simulink model "FunctionalArchitecture"  (R2020b)
settings: Solver=VariableStepAuto  StartTime=0.0  StopTime=10.0  RelTol=1e-3
settings Model: Creator=jantonio  LastModifiedBy=jantonio

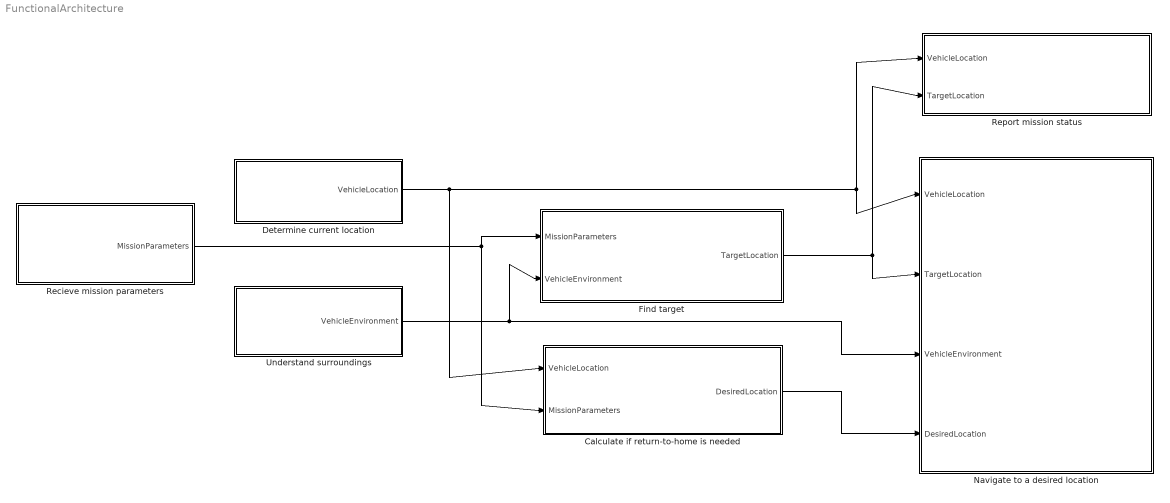
== system FunctionalArchitecture ==
  Calculate if return-to-home is needed : Subsystem
      settings: PortSchema="{\"entries\":[{\"content\":{\"headerSize\":26,\"margin\":15,\"minimumSpacing\":25,\"sides\":[{\"content\":{\"connectorIds\":[\"In2\",\"In1\"]},\"type\":\"ConnectorPlacement.EquallySpacedRectSide\",\"uuid\":\"39ab5f6e-200b-418c-957c-0427e0a2d192\"},{\"content\":{\"connectorIds\":[\"Out1\"],\"side\":\"RIGHT\"},\"type\":\"ConnectorPlacement.EquallySpacedRectSide\",\"uuid\":\"2abcd6b7-9ef0-4689-b904-6f1a8a48cdb7\"},{\"content\":{\"connectorIds\":[],\"side\":\"TOP\"},\"type\":\"ConnectorPlacement.EquallySpacedRectSide\",\"uuid\":\"3ddcf8bd-fb65-4c69-ae6b-4c30928b7beb\"}]},\"type\":\"ConnectorPlacement.EquallySpacedConnector\",\"uuid\":\"ab0c7103-d8ef-4055-8653-3cf105b5edbd\"}],\"packageUris\":[\"http://schema.mathworks.com/mf0/Connector/19700101\"],\"version\":\"1.0\"}"
  Determine current location : Subsystem
      settings: PortSchema="{\"entries\":[{\"content\":{\"headerSize\":26,\"margin\":15,\"minimumSpacing\":25,\"sides\":[{\"content\":{\"connectorIds\":[]},\"type\":\"ConnectorPlacement.EquallySpacedRectSide\",\"uuid\":\"39ab5f6e-200b-418c-957c-0427e0a2d192\"},{\"content\":{\"connectorIds\":[\"Out1\"],\"side\":\"RIGHT\"},\"type\":\"ConnectorPlacement.EquallySpacedRectSide\",\"uuid\":\"2abcd6b7-9ef0-4689-b904-6f1a8a48cdb7\"},{\"content\":{\"connectorIds\":[],\"side\":\"TOP\"},\"type\":\"ConnectorPlacement.EquallySpacedRectSide\",\"uuid\":\"3ddcf8bd-fb65-4c69-ae6b-4c30928b7beb\"}]},\"type\":\"ConnectorPlacement.EquallySpacedConnector\",\"uuid\":\"ab0c7103-d8ef-4055-8653-3cf105b5edbd\"}],\"packageUris\":[\"http://schema.mathworks.com/mf0/Connector/19700101\"],\"version\":\"1.0\"}"
  Find target : Subsystem
      settings: PortSchema="{\"entries\":[{\"content\":{\"headerSize\":26,\"margin\":15,\"minimumSpacing\":25,\"sides\":[{\"content\":{\"connectorIds\":[\"In1\",\"In2\"]},\"type\":\"ConnectorPlacement.EquallySpacedRectSide\",\"uuid\":\"39ab5f6e-200b-418c-957c-0427e0a2d192\"},{\"content\":{\"connectorIds\":[\"Out1\"],\"side\":\"RIGHT\"},\"type\":\"ConnectorPlacement.EquallySpacedRectSide\",\"uuid\":\"2abcd6b7-9ef0-4689-b904-6f1a8a48cdb7\"},{\"content\":{\"connectorIds\":[],\"side\":\"TOP\"},\"type\":\"ConnectorPlacement.EquallySpacedRectSide\",\"uuid\":\"3ddcf8bd-fb65-4c69-ae6b-4c30928b7beb\"}]},\"type\":\"ConnectorPlacement.EquallySpacedConnector\",\"uuid\":\"ab0c7103-d8ef-4055-8653-3cf105b5edbd\"}],\"packageUris\":[\"http://schema.mathworks.com/mf0/Connector/19700101\"],\"version\":\"1.0\"}"
  Navigate to a desired location : Subsystem
      settings: PortSchema="{\"entries\":[{\"content\":{\"headerSize\":26,\"margin\":15,\"minimumSpacing\":25,\"sides\":[{\"content\":{\"connectorIds\":[\"In3\",\"In2\",\"In4\",\"In1\"]},\"type\":\"ConnectorPlacement.EquallySpacedRectSide\",\"uuid\":\"39ab5f6e-200b-418c-957c-0427e0a2d192\"},{\"content\":{\"connectorIds\":[],\"side\":\"RIGHT\"},\"type\":\"ConnectorPlacement.EquallySpacedRectSide\",\"uuid\":\"2abcd6b7-9ef0-4689-b904-6f1a8a48cdb7\"},{\"content\":{\"connectorIds\":[],\"side\":\"TOP\"},\"type\":\"ConnectorPlacement.EquallySpacedRectSide\",\"uuid\":\"3ddcf8bd-fb65-4c69-ae6b-4c30928b7beb\"}]},\"type\":\"ConnectorPlacement.EquallySpacedConnector\",\"uuid\":\"ab0c7103-d8ef-4055-8653-3cf105b5edbd\"}],\"packageUris\":[\"http://schema.mathworks.com/mf0/Connector/19700101\"],\"version\":\"1.0\"}"
  Recieve mission parameters : Subsystem
      settings: PortSchema="{\"entries\":[{\"content\":{\"headerSize\":26,\"margin\":15,\"minimumSpacing\":25,\"sides\":[{\"content\":{\"connectorIds\":[]},\"type\":\"ConnectorPlacement.EquallySpacedRectSide\",\"uuid\":\"39ab5f6e-200b-418c-957c-0427e0a2d192\"},{\"content\":{\"connectorIds\":[\"Out1\"],\"side\":\"RIGHT\"},\"type\":\"ConnectorPlacement.EquallySpacedRectSide\",\"uuid\":\"2abcd6b7-9ef0-4689-b904-6f1a8a48cdb7\"},{\"content\":{\"connectorIds\":[],\"side\":\"TOP\"},\"type\":\"ConnectorPlacement.EquallySpacedRectSide\",\"uuid\":\"3ddcf8bd-fb65-4c69-ae6b-4c30928b7beb\"}]},\"type\":\"ConnectorPlacement.EquallySpacedConnector\",\"uuid\":\"ab0c7103-d8ef-4055-8653-3cf105b5edbd\"}],\"packageUris\":[\"http://schema.mathworks.com/mf0/Connector/19700101\"],\"version\":\"1.0\"}"
  Report mission status : Subsystem
      settings: PortSchema="{\"entries\":[{\"content\":{\"headerSize\":26,\"margin\":15,\"minimumSpacing\":25,\"sides\":[{\"content\":{\"connectorIds\":[\"In2\",\"In1\"]},\"type\":\"ConnectorPlacement.EquallySpacedRectSide\",\"uuid\":\"39ab5f6e-200b-418c-957c-0427e0a2d192\"},{\"content\":{\"connectorIds\":[],\"side\":\"RIGHT\"},\"type\":\"ConnectorPlacement.EquallySpacedRectSide\",\"uuid\":\"2abcd6b7-9ef0-4689-b904-6f1a8a48cdb7\"},{\"content\":{\"connectorIds\":[],\"side\":\"TOP\"},\"type\":\"ConnectorPlacement.EquallySpacedRectSide\",\"uuid\":\"3ddcf8bd-fb65-4c69-ae6b-4c30928b7beb\"}]},\"type\":\"ConnectorPlacement.EquallySpacedConnector\",\"uuid\":\"ab0c7103-d8ef-4055-8653-3cf105b5edbd\"}],\"packageUris\":[\"http://schema.mathworks.com/mf0/Connector/19700101\"],\"version\":\"1.0\"}"
  Understand surroundings : Subsystem
      settings: PortSchema="{\"entries\":[{\"content\":{\"headerSize\":26,\"margin\":15,\"minimumSpacing\":25,\"sides\":[{\"content\":{\"connectorIds\":[]},\"type\":\"ConnectorPlacement.EquallySpacedRectSide\",\"uuid\":\"39ab5f6e-200b-418c-957c-0427e0a2d192\"},{\"content\":{\"connectorIds\":[\"Out1\"],\"side\":\"RIGHT\"},\"type\":\"ConnectorPlacement.EquallySpacedRectSide\",\"uuid\":\"2abcd6b7-9ef0-4689-b904-6f1a8a48cdb7\"},{\"content\":{\"connectorIds\":[],\"side\":\"TOP\"},\"type\":\"ConnectorPlacement.EquallySpacedRectSide\",\"uuid\":\"3ddcf8bd-fb65-4c69-ae6b-4c30928b7beb\"}]},\"type\":\"ConnectorPlacement.EquallySpacedConnector\",\"uuid\":\"ab0c7103-d8ef-4055-8653-3cf105b5edbd\"}],\"packageUris\":[\"http://schema.mathworks.com/mf0/Connector/19700101\"],\"version\":\"1.0\"}"
  wires:
  Find target/1(TargetLocation) -> Report mission status/1(TargetLocation), Navigate to a desired location/2(TargetLocation)
  Understand surroundings/1(VehicleEnvironment) -> Find target/2(VehicleEnvironment), Navigate to a desired location/4(VehicleEnvironment)
  Determine current location/1(VehicleLocation) -> Calculate if return-to-home is needed/2(VehicleLocation), Report mission status/2(VehicleLocation), Navigate to a desired location/3(VehicleLocation)
  Recieve mission parameters/1(MissionParameters) -> Calculate if return-to-home is needed/1(MissionParameters), Find target/1(MissionParameters)
  Calculate if return-to-home is needed/1(DesiredLocation) -> Navigate to a desired location/1(DesiredLocation)

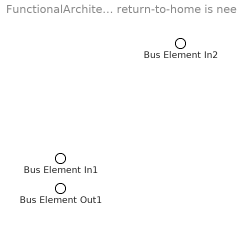
== system FunctionalArchitecture/Calculate if return-to-home is needed ==
  Bus Element In2 : Inport  PortName=MissionParameters
  Bus Element In1 : Inport  Port=2  PortName=VehicleLocation
  Bus Element Out1 : Outport  PortName=DesiredLocation

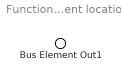
== system FunctionalArchitecture/Determine current location ==
  Bus Element Out1 : Outport  PortName=VehicleLocation

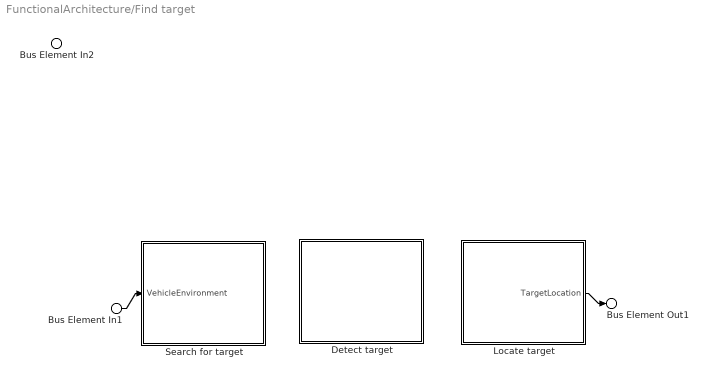
== system FunctionalArchitecture/Find target ==
  Bus Element In2 : Inport  PortName=MissionParameters
  Bus Element In1 : Inport  Port=2  PortName=VehicleEnvironment
  Detect target : Subsystem
      settings: PortSchema="{\"entries\":[{\"content\":{\"headerSize\":26,\"margin\":15,\"minimumSpacing\":25,\"sides\":[{\"content\":{\"connectorIds\":[]},\"type\":\"ConnectorPlacement.EquallySpacedRectSide\",\"uuid\":\"39ab5f6e-200b-418c-957c-0427e0a2d192\"},{\"content\":{\"connectorIds\":[],\"side\":\"RIGHT\"},\"type\":\"ConnectorPlacement.EquallySpacedRectSide\",\"uuid\":\"2abcd6b7-9ef0-4689-b904-6f1a8a48cdb7\"},{\"content\":{\"connectorIds\":[],\"side\":\"TOP\"},\"type\":\"ConnectorPlacement.EquallySpacedRectSide\",\"uuid\":\"3ddcf8bd-fb65-4c69-ae6b-4c30928b7beb\"}]},\"type\":\"ConnectorPlacement.EquallySpacedConnector\",\"uuid\":\"ab0c7103-d8ef-4055-8653-3cf105b5edbd\"}],\"packageUris\":[\"http://schema.mathworks.com/mf0/Connector/19700101\"],\"version\":\"1.0\"}"
  Locate target : Subsystem
      settings: PortSchema="{\"entries\":[{\"content\":{\"headerSize\":26,\"margin\":15,\"minimumSpacing\":25,\"sides\":[{\"content\":{\"connectorIds\":[]},\"type\":\"ConnectorPlacement.EquallySpacedRectSide\",\"uuid\":\"39ab5f6e-200b-418c-957c-0427e0a2d192\"},{\"content\":{\"connectorIds\":[\"Out1\"],\"side\":\"RIGHT\"},\"type\":\"ConnectorPlacement.EquallySpacedRectSide\",\"uuid\":\"2abcd6b7-9ef0-4689-b904-6f1a8a48cdb7\"},{\"content\":{\"connectorIds\":[],\"side\":\"TOP\"},\"type\":\"ConnectorPlacement.EquallySpacedRectSide\",\"uuid\":\"3ddcf8bd-fb65-4c69-ae6b-4c30928b7beb\"}]},\"type\":\"ConnectorPlacement.EquallySpacedConnector\",\"uuid\":\"ab0c7103-d8ef-4055-8653-3cf105b5edbd\"}],\"packageUris\":[\"http://schema.mathworks.com/mf0/Connector/19700101\"],\"version\":\"1.0\"}"
  Search for target : Subsystem
      settings: PortSchema="{\"entries\":[{\"content\":{\"headerSize\":26,\"margin\":15,\"minimumSpacing\":25,\"sides\":[{\"content\":{\"connectorIds\":[\"In1\"]},\"type\":\"ConnectorPlacement.EquallySpacedRectSide\",\"uuid\":\"39ab5f6e-200b-418c-957c-0427e0a2d192\"},{\"content\":{\"connectorIds\":[],\"side\":\"RIGHT\"},\"type\":\"ConnectorPlacement.EquallySpacedRectSide\",\"uuid\":\"2abcd6b7-9ef0-4689-b904-6f1a8a48cdb7\"},{\"content\":{\"connectorIds\":[],\"side\":\"TOP\"},\"type\":\"ConnectorPlacement.EquallySpacedRectSide\",\"uuid\":\"3ddcf8bd-fb65-4c69-ae6b-4c30928b7beb\"}]},\"type\":\"ConnectorPlacement.EquallySpacedConnector\",\"uuid\":\"ab0c7103-d8ef-4055-8653-3cf105b5edbd\"}],\"packageUris\":[\"http://schema.mathworks.com/mf0/Connector/19700101\"],\"version\":\"1.0\"}"
  Bus Element Out1 : Outport  PortName=TargetLocation
  wires:
  Bus Element In1/1 -> Search for target/1(VehicleEnvironment)
  Locate target/1(TargetLocation) -> Bus Element Out1/1

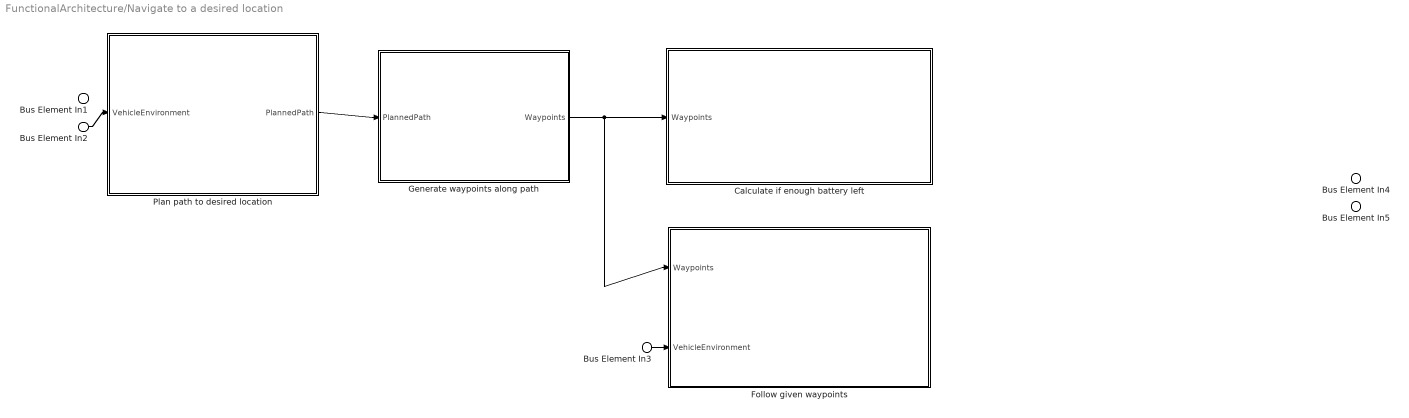
== system FunctionalArchitecture/Navigate to a desired location ==
  Bus Element In5 : Inport  PortName=DesiredLocation
  Bus Element In1 : Inport  Port=2  PortName=TargetLocation
  Bus Element In4 : Inport  Port=3  PortName=VehicleLocation
  Bus Element In3 : Inport  Port=4  PortName=VehicleEnvironment
  Bus Element In2 : Inport  Port=4  PortName=VehicleEnvironment
  Calculate if enough battery left : Subsystem
      settings: PortSchema="{\"entries\":[{\"content\":{\"headerSize\":26,\"margin\":15,\"minimumSpacing\":25,\"sides\":[{\"content\":{\"connectorIds\":[\"In1\"]},\"type\":\"ConnectorPlacement.EquallySpacedRectSide\",\"uuid\":\"39ab5f6e-200b-418c-957c-0427e0a2d192\"},{\"content\":{\"connectorIds\":[],\"side\":\"RIGHT\"},\"type\":\"ConnectorPlacement.EquallySpacedRectSide\",\"uuid\":\"2abcd6b7-9ef0-4689-b904-6f1a8a48cdb7\"},{\"content\":{\"connectorIds\":[],\"side\":\"TOP\"},\"type\":\"ConnectorPlacement.EquallySpacedRectSide\",\"uuid\":\"3ddcf8bd-fb65-4c69-ae6b-4c30928b7beb\"}]},\"type\":\"ConnectorPlacement.EquallySpacedConnector\",\"uuid\":\"ab0c7103-d8ef-4055-8653-3cf105b5edbd\"}],\"packageUris\":[\"http://schema.mathworks.com/mf0/Connector/19700101\"],\"version\":\"1.0\"}"
  Follow given waypoints : Subsystem
      settings: PortSchema="{\"entries\":[{\"content\":{\"headerSize\":26,\"margin\":15,\"minimumSpacing\":25,\"sides\":[{\"content\":{\"connectorIds\":[\"In1\",\"In2\"]},\"type\":\"ConnectorPlacement.EquallySpacedRectSide\",\"uuid\":\"39ab5f6e-200b-418c-957c-0427e0a2d192\"},{\"content\":{\"connectorIds\":[],\"side\":\"RIGHT\"},\"type\":\"ConnectorPlacement.EquallySpacedRectSide\",\"uuid\":\"2abcd6b7-9ef0-4689-b904-6f1a8a48cdb7\"},{\"content\":{\"connectorIds\":[],\"side\":\"TOP\"},\"type\":\"ConnectorPlacement.EquallySpacedRectSide\",\"uuid\":\"3ddcf8bd-fb65-4c69-ae6b-4c30928b7beb\"}]},\"type\":\"ConnectorPlacement.EquallySpacedConnector\",\"uuid\":\"ab0c7103-d8ef-4055-8653-3cf105b5edbd\"}],\"packageUris\":[\"http://schema.mathworks.com/mf0/Connector/19700101\"],\"version\":\"1.0\"}"
  Generate waypoints along path : Subsystem
      settings: PortSchema="{\"entries\":[{\"content\":{\"headerSize\":26,\"margin\":15,\"minimumSpacing\":25,\"sides\":[{\"content\":{\"connectorIds\":[\"In1\"]},\"type\":\"ConnectorPlacement.EquallySpacedRectSide\",\"uuid\":\"39ab5f6e-200b-418c-957c-0427e0a2d192\"},{\"content\":{\"connectorIds\":[\"Out1\"],\"side\":\"RIGHT\"},\"type\":\"ConnectorPlacement.EquallySpacedRectSide\",\"uuid\":\"2abcd6b7-9ef0-4689-b904-6f1a8a48cdb7\"},{\"content\":{\"connectorIds\":[],\"side\":\"TOP\"},\"type\":\"ConnectorPlacement.EquallySpacedRectSide\",\"uuid\":\"3ddcf8bd-fb65-4c69-ae6b-4c30928b7beb\"}]},\"type\":\"ConnectorPlacement.EquallySpacedConnector\",\"uuid\":\"ab0c7103-d8ef-4055-8653-3cf105b5edbd\"}],\"packageUris\":[\"http://schema.mathworks.com/mf0/Connector/19700101\"],\"version\":\"1.0\"}"
  Plan path to desired location : Subsystem
      settings: PortSchema="{\"entries\":[{\"content\":{\"headerSize\":26,\"margin\":15,\"minimumSpacing\":25,\"sides\":[{\"content\":{\"connectorIds\":[\"In1\"]},\"type\":\"ConnectorPlacement.EquallySpacedRectSide\",\"uuid\":\"39ab5f6e-200b-418c-957c-0427e0a2d192\"},{\"content\":{\"connectorIds\":[\"Out1\"],\"side\":\"RIGHT\"},\"type\":\"ConnectorPlacement.EquallySpacedRectSide\",\"uuid\":\"2abcd6b7-9ef0-4689-b904-6f1a8a48cdb7\"},{\"content\":{\"connectorIds\":[],\"side\":\"TOP\"},\"type\":\"ConnectorPlacement.EquallySpacedRectSide\",\"uuid\":\"3ddcf8bd-fb65-4c69-ae6b-4c30928b7beb\"}]},\"type\":\"ConnectorPlacement.EquallySpacedConnector\",\"uuid\":\"ab0c7103-d8ef-4055-8653-3cf105b5edbd\"}],\"packageUris\":[\"http://schema.mathworks.com/mf0/Connector/19700101\"],\"version\":\"1.0\"}"
  wires:
  Plan path to desired location/1(PlannedPath) -> Generate waypoints along path/1(PlannedPath)
  Generate waypoints along path/1(Waypoints) -> Follow given waypoints/1(Waypoints), Calculate if enough battery left/1(Waypoints)
  Bus Element In3/1 -> Follow given waypoints/2(VehicleEnvironment)
  Bus Element In2/1 -> Plan path to desired location/1(VehicleEnvironment)

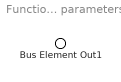
== system FunctionalArchitecture/Recieve mission parameters ==
  Bus Element Out1 : Outport  PortName=MissionParameters

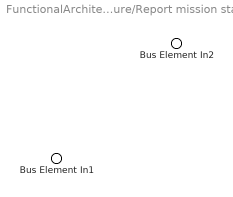
== system FunctionalArchitecture/Report mission status ==
  Bus Element In2 : Inport  PortName=TargetLocation
  Bus Element In1 : Inport  Port=2  PortName=VehicleLocation

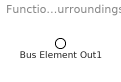
== system FunctionalArchitecture/Understand surroundings ==
  Bus Element Out1 : Outport  PortName=VehicleEnvironment

== system FunctionalArchitecture/Find target/Detect target ==

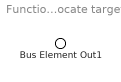
== system FunctionalArchitecture/Find target/Locate target ==
  Bus Element Out1 : Outport  PortName=TargetLocation

== system FunctionalArchitecture/Find target/Search for target ==
  Bus Element In1 : Inport  PortName=VehicleEnvironment

== system FunctionalArchitecture/Navigate to a desired location/Calculate if enough battery left ==
  Bus Element In1 : Inport  PortName=Waypoints

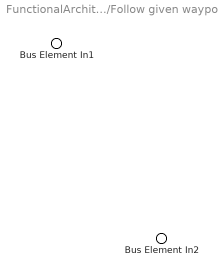
== system FunctionalArchitecture/Navigate to a desired location/Follow given waypoints ==
  Bus Element In1 : Inport  PortName=Waypoints
  Bus Element In2 : Inport  Port=2  PortName=VehicleEnvironment

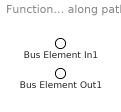
== system FunctionalArchitecture/Navigate to a desired location/Generate waypoints along path ==
  Bus Element In1 : Inport  PortName=PlannedPath
  Bus Element Out1 : Outport  PortName=Waypoints

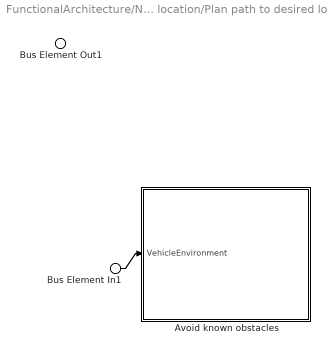
== system FunctionalArchitecture/Navigate to a desired location/Plan path to desired location ==
  Bus Element In1 : Inport  PortName=VehicleEnvironment
  Avoid known obstacles : Subsystem
      settings: PortSchema="{\"entries\":[{\"content\":{\"headerSize\":26,\"margin\":15,\"minimumSpacing\":25,\"sides\":[{\"content\":{\"connectorIds\":[\"In1\"]},\"type\":\"ConnectorPlacement.EquallySpacedRectSide\",\"uuid\":\"39ab5f6e-200b-418c-957c-0427e0a2d192\"},{\"content\":{\"connectorIds\":[],\"side\":\"RIGHT\"},\"type\":\"ConnectorPlacement.EquallySpacedRectSide\",\"uuid\":\"2abcd6b7-9ef0-4689-b904-6f1a8a48cdb7\"},{\"content\":{\"connectorIds\":[],\"side\":\"TOP\"},\"type\":\"ConnectorPlacement.EquallySpacedRectSide\",\"uuid\":\"3ddcf8bd-fb65-4c69-ae6b-4c30928b7beb\"}]},\"type\":\"ConnectorPlacement.EquallySpacedConnector\",\"uuid\":\"ab0c7103-d8ef-4055-8653-3cf105b5edbd\"}],\"packageUris\":[\"http://schema.mathworks.com/mf0/Connector/19700101\"],\"version\":\"1.0\"}"
  Bus Element Out1 : Outport  PortName=PlannedPath
  wires:
  Bus Element In1/1 -> Avoid known obstacles/1(VehicleEnvironment)

== system FunctionalArchitecture/Navigate to a desired location/Plan path to desired location/Avoid known obstacles ==
  Bus Element In1 : Inport  PortName=VehicleEnvironment
